simulink model "prototipo"  (R2022b)
settings: Solver=ode3  StartTime=0.0  StopTime=10  RelTol=1e-3  EnableMultiTasking=on
model workspace (MAT data in the model file):
  RGBData = [62 63 65 64 60 62 65 62 60 59 59 59 ... (230400 elements, 320x240x3)]
libraries: sensehatlib x2, raspberrypiAVlib x2, visionanalysis x1, visiontextngfix x1
(part 1 of 2)
settings Model: FPTRunName=Active  ExtModeTrigDuration=2  Creator=alber  LastModifiedBy=alber
settings SolverCC: AlgebraicLoopSolver=TrustRegion  PositivePriorityOrder=on
settings DataIOCC: LimitDataPoints=on  SaveFormat=Array
settings OptimizationCC: ExpressionDepthLimit=2147483647  ZeroExternalMemoryAtStartup=off  ZeroInternalMemoryAtStartup=off  LifeSpan=Inf  MaxStackSize=64
settings DebuggingCC: UnderspecifiedInitializationDetection=Classic  MergeDetectMultiDrivingBlocksExec=none  FcnCallInpInsideContextMsg=warning  UnconnectedInputMsg=warning  UnconnectedOutputMsg=warning  UnconnectedLineMsg=warning  AllowSymbolicDim=off  StateNameClashWarn=warning  SFUnexpectedBacktrackingDiag=warning  SFNoUnconditionalDefaultTransitionDiag=warning  SFExecutionAtInitializationDiag=none  SFMachineParentedDataDiag=warning  ArithmeticOperatorsInVariantConditions=warning
settings HardwareCC: ProdBitPerPointer=32  ProdBitPerSizeT=32  ProdBitPerPtrDiffT=32  ProdLargestAtomicInteger=Long  ProdLargestAtomicFloat=Double  ProdWordSize=32  ProdHWDeviceType=ARM Compatible->ARM Cortex  UseEmbeddedCoderFeatures=off
settings ModelReferenceCC: EnableRefExpFcnMdlSchedulingChecks=on  PropagateSignalLabelsOutOfModel=off
settings SFSimCC: SimUseLocalCustomCode=off  CustomCodeUndefinedFunction=UseInterfaceOnly
settings RTWCC: Description=Embedded Coder  SystemTargetFile=ert.tlc  HardwareBoard=Raspberry Pi  TemplateMakefile=ert_default_tmf  RTWVerbose=off  RTWUseLocalCustomCode=off  Toolchain=GNU GCC Embedded Linux  BuildConfiguration=Faster Runs  TargetLang=C++  DLTargetLibrary=arm-compute  DLArmComputeVersion=19.05  DLArmComputeArch=armv7
settings CodeAppCC: StateflowObjectComments=on
settings ERTTargetCC: TargetLangStandard=C++03 (ISO)  MultiwordLength=2048  ERTCustomFileBanners=off  CodeInterfacePackaging=C++ class  SupportContinuousTime=on  SupportNonInlinedSFcns=on  RemoveResetFunc=off  SupportVariableSizeSignals=on  ModelStepFunctionPrototypeControlCompliant=off  ConvertIfToSwitch=off  SuppressUnreachableDefaultCases=off
settings ConfigComp: CovMetricSettings=dw  CovSaveCumulativeToWorkspaceVar=on  CovSaveSingleToWorkspaceVar=on  CovExternalEMLEnable=off  CovSFcnEnable=off

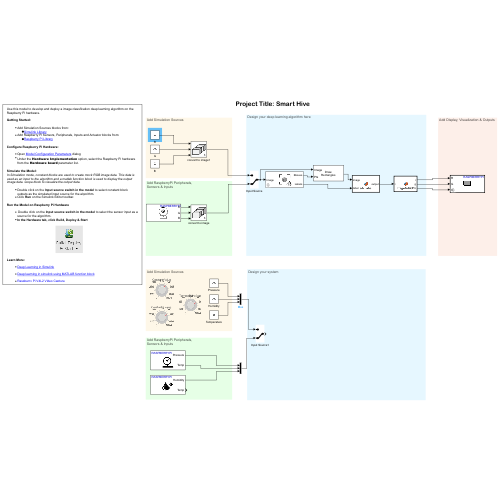
[thumbnail: Simulink's stored preview of the top-level diagram]
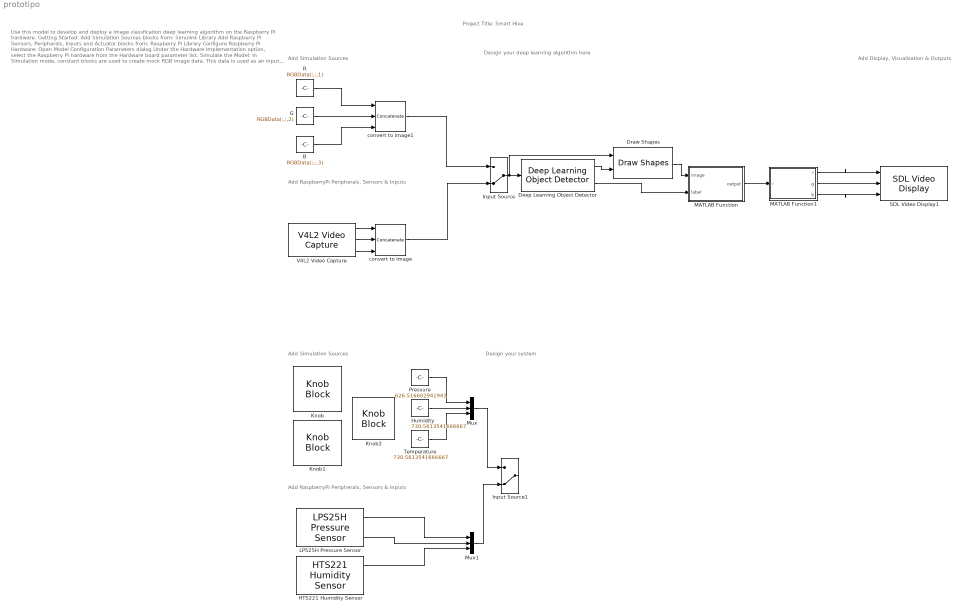
== system prototipo ==
  note: Use this model to develop and deploy a image classfication deep learning algorithm on the Raspberry Pi hardware.
      |
      | Getting Started:
      |
      | Add Simulation Sources blocks from:
      | Simulink Library
      | Add Raspberry Pi Sensors, Peripherals, Inputs and Actuator blocks from:
      | Raspberry Pi Library
      |
      | Configure Raspberry Pi Hardware:
      |
      | Open Model Configuration Parameters dialog
      | Under the Hardware Implementation option, select the Raspberry Pi hardware from the Hardware board parameter list.
      |
      | Simulate the Model:
      | In Simulation mode, constant blocks are used to create mock RGB image data. This data is used as an input to the algorithm and a matlab function block is used to display the output image data. scope block to visualize the output data.
      |
      | Double click on the Input source switch in the model to select constant block outputs as the simulated input source for the algorithm.
      | Click Run on the Simulink Editor toolbar.
      |
      | Run the Model on Raspberry Pi Hardware
      |
      | Double click on the Input source switch in the model to select the sensor input as a source for the algorithm.
      | In the Hardware tab, click Build, Deploy & Start
      |
      | Learn More:
      |
      | Deep Learning in Simulink
      | Deep learning in simulink using MATLAB function block
      | Raspberry Pi V4L2 Video Capture
      | Raspberry Pi SDL Video Display
  note: Add Display, Visualization & Outputs
  note: Add Simulation Sources
  note: Project Title: Smart Hive
  note: Design your deep learning algorithm here
  note: Add RaspberryPi Peripherals,
      | Sensors & Inputs
  note: Add Simulation Sources
  note: Add RaspberryPi Peripherals,
      | Sensors & Inputs
  note: Design your system
  B : Constant  Value=RGBData(:,:,3)  OutDataTypeStr=uint8  SampleTime=0.1
  Deep Learning Object Detector : visionanalysis/Deep Learning Object Detector  Detector=Detector from MAT-file  DetectorFunction=untitled  DetectorFilePath=untitled.mat  MaxDetections=500  Bboxes=on  Scores=off  UseROI=off  ROI=[1 1 100 100]  Threshold=0.5  NumStrongestRegions=2000  UseMinSize=off  MinSize=[1 1]  UseMaxSize=off  MaxSize=[50 50]  ForceInterpretedSim=off
  Draw Shapes : visiontextngfix/Draw Shapes  shape=Rectangles  fill=off  lineWidth=1  fillClrSource=Specify via dialog  display=Black  intensity=200  color=[200 255 100]  opacity=0.6  viewport=Entire image  antialiasing=off  inType=Obsolete  imagePorts=One multidimensional signal  roundingMode=Floor  overflowMode=off  memoryMode=Specify word length  memoryWordLength=16  prodOutputMode=Binary point scaling  prodOutputWordLength=32  prodOutputFracLength=14  memoryFracLength=15
  G : Constant  Value=RGBData(:,:,2)  OutDataTypeStr=uint8  SampleTime=0.1
  HTS221 Humidity Sensor : sensehatlib/HTS221 Humidity Sensor  BoardProperty=Pi 2 Model B  OutputDataRate=12.5 Hz  SampleTime=0.1
  Humidity : Constant  Value=730.5613541666667
  Input Source : ManualSwitch  CurrentSetting=0
  Input Source1 : ManualSwitch  CurrentSetting=0
  Knob : KnobBlock  ScaleMax=1024
  Knob1 : KnobBlock  ScaleMax=1024
  Knob2 : KnobBlock  ScaleMax=1024
  LPS25H Pressure Sensor : sensehatlib/LPS25H Pressure Sensor  BoardProperty=Pi 2 Model B  OutputDataRate=25 Hz  SampleTime=0.1
  MATLAB Function : MATLAB Function  TreatAsAtomicUnit=on
  MATLAB Function1 : MATLAB Function  TreatAsAtomicUnit=on
  Mux : Mux  Inputs=3
  Mux1 : Mux  Inputs=3
  Pressure : Constant  Value=626.516602941941
  R : Constant  Value=RGBData(:,:,1)  OutDataTypeStr=uint8  SampleTime=0.1
  SDL Video Display1 : raspberrypiAVlib/SDL Video Display  title=SDL Video Display  pixelFormat=RGB  pixelOrder=Planar  rowMajor=on  blockPlatform=Raspberry Pi
  Temperature : Constant  Value=730.5613541666667
  V4L2 Video Capture : raspberrypiAVlib/V4L2 Video Capture  DeviceName=/dev/video0  Resolution=320x240  CustomResolution=[ 320, 240 ]  PixelFormat=RGB  SampleTime=0.1  pixelOrder=planar  simOutput=Colorbars  imSizeSelection=320x240  imSize=[640, 480]  roi=[0, 0, 640, 480]  m_devName='/dev/video0'  blockPlatform=LINUX  HorizontalFlip=off  VerticalFlip=off  Brightness=0.5  Saturation=0.5  Contrast=0.5  Sharpness=0.5  CameraPan=0  CameraTilt=0  CameraZoom=0.5  EnableManualFocus=on  ManualFocus=0.5
  convert to image : Concatenate  NumInputs=3  Mode=Multidimensional array  ConcatenateDimension=3
  convert to image1 : Concatenate  NumInputs=3  Mode=Multidimensional array  ConcatenateDimension=3
  wires:
  Input Source/1 -> Draw Shapes/1, Deep Learning Object Detector/1
  MATLAB Function1/2(g) -> SDL Video Display1/2
  MATLAB Function1/1(r) -> SDL Video Display1/1
  MATLAB Function1/3(b) -> SDL Video Display1/3
  R/1 -> convert to image1/1
  G/1 -> convert to image1/2
  B/1 -> convert to image1/3
  V4L2 Video Capture/2 -> convert to image/2
  V4L2 Video Capture/1 -> convert to image/1
  V4L2 Video Capture/3 -> convert to image/3
  convert to image1/1 -> Input Source/1
  convert to image/1 -> Input Source/2
  Deep Learning Object Detector/1 -> Draw Shapes/2
  Draw Shapes/1 -> MATLAB Function/1(image)
  Deep Learning Object Detector/2 -> MATLAB Function/2(label)
  MATLAB Function/1(output) -> MATLAB Function1/1(i)
  Pressure/1 -> Mux/1
  Humidity/1 -> Mux/2
  Temperature/1 -> Mux/3
  LPS25H Pressure Sensor/1 -> Mux1/1
  HTS221 Humidity Sensor/1 -> Mux1/3
  LPS25H Pressure Sensor/2 -> Mux1/2
  Mux/1 -> Input Source1/1
  Mux1/1 -> Input Source1/2
